simulink model "BPM_HA_Spin_sfun_xk"  (R2022b)
settings: configuration reference "ModelConfig_var" (kept outside this file)
InitFcn:
  | %% BUS initialization
  | Xabc.A = 0;
  | Xabc.B = 0;
  | Xabc.C = 0;
  | % -------------------------------------------------------------------------
  | Simulink.Bus.createObject(Xabc)
  | XabcBus = slBus1;
  | clear slBus1
  | 
  | %% Parameter Structure initialization
  | Motor_prm_init_bpm;
model workspace (MAT data in the model file):
  Mech_HAs_CF = 0
  Mech_HAs_J_drum = 0
  Mech_HAs_TR = 0
  Mech_HAs_damp = 0
  Mech_HAs_m_unb = 0
  Mech_HAs_r_unb = 0
  Mech_VAa_J_basket = 0
  Mech_VAa_J_impeller = 0
  Mech_VAa_basket_dens = 0
  Mech_VAa_basket_dia = 0
  Mech_VAa_belt_ratio = 0
  Mech_VAa_clothes_mass = 0
  Mech_VAa_gear_ratio = 0
  Mech_VAa_imp_dens = 0
  Mech_VAa_water_vol = 0
  Mech_VAs_D_r = 0
  Mech_VAs_I_zt = 0
  Mech_VAs_K = 2700
  Mech_VAs_T_f = 0
  Mech_VAs_belt_rat = 0
  Mech_VAs_d = 0
  Mech_VAs_e = 0
  Mech_VAs_m_b1 = 0
  Mech_VAs_m_b2 = 0
  Mech_VAs_m_d = 0
  Mech_VAs_m_t = 0
  Mech_VAs_m_u = 0
  Time_step = 0.0001
  Time_step_solver = 0
  bpm_B = 0
  bpm_Ipk = [0 1 2 3 4 5 6 7]
  bpm_Jrotor = 0
  bpm_Ld_0 = 0.02117
  bpm_Ld_a = [0.02117 0.02117 0.02117 0.02117 0.02117 0.02117 0.02117 0.02117]
  bpm_Loss_Power = [0 1 2 3 4 5 6 7]
  bpm_Loss_Speed = [0 1 2 3 4 5 6 7]
  bpm_Loss_flag = 1
  bpm_Loss_th = 10
  bpm_Lq_0 = 0.02117
  bpm_Lq_b = [0.02117 0.02117 0.02117 0.02117 0.02117 0.02117 0.02117 0.02117]
  bpm_Ls_sat_flag = 1
  bpm_NPP = 0
  bpm_PM_flux_h1_0 = 0
  bpm_PM_rotor_alpha = 0
  bpm_Rs_0 = 0
  bpm_Rs_stator_alpha = 0
  bpm_Rsa_aux = 0
  bpm_Rsb_aux = 0
  bpm_Rsc_aux = 0
  bpm_TR = 1
  bpm_Temp_rotor_0 = 0
  bpm_Temp_stator_0 = 0
libraries: bpm_dq_S_noH_D_RL_U_HA_Spin_xk x1
settings Model: ParameterArgumentNames=Mech_HAs_CF,Mech_HAs_J_drum,Mech_HAs_TR,Mech_HAs_damp,Mech_HAs_m_unb,Mech_HAs_r_unb,Mech_VAa_J_basket,Mech_VAa_J_impeller,Mech_VAa_basket_dens,Mech_VAa_basket_dia,Mech_VAa_belt_ratio,Mech_VAa_clothes_mass,Mech_VAa_gear_ratio,Mech_VAa_imp_dens,Mech_VAa_water_vol,Mech_VAs_D_r,Mech_VAs_I_zt,Mech_VAs_K,Mech_VAs_T_f,Mech_VAs_belt_rat,Mech_VAs_d,Mech_VAs_e,Mech_VAs_m_b1,Mech_VAs_m_b2,Mech_VAs_m_d,Mech_VAs_m_t,Mech_VAs_m_u,Time_step_solver,bpm_B,bpm_Ipk,bpm_Jrotor,bpm_Ld_0,bpm_Ld_a,bpm_Loss_Power,bpm_Loss_Speed,bpm_Loss_flag,bpm_Loss_th,bpm_Lq_0,bpm_Lq_b,bpm_Ls_sat_flag,bpm_NPP,bpm_PM_flux_h1_0,bpm_PM_rotor_alpha,bpm_Rs_0,bpm_Rs_stator_alpha,bpm_Rsa_aux,bpm_Rsb_aux,bpm_Rsc_aux,bpm_TR,bpm_Temp_rotor_0,bpm_Temp_stator_0  Creator=BEDNASA  LastModifiedBy=BEDNASA
settings ConfigSetRef: SourceName=ModelConfig_var  SourceLocation=Base Workspace

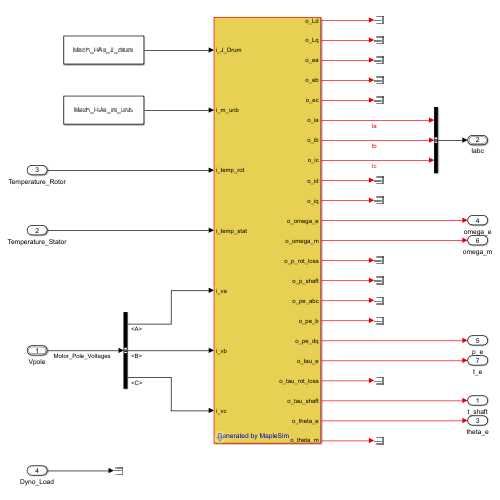
[thumbnail: Simulink's stored preview of the top-level diagram]
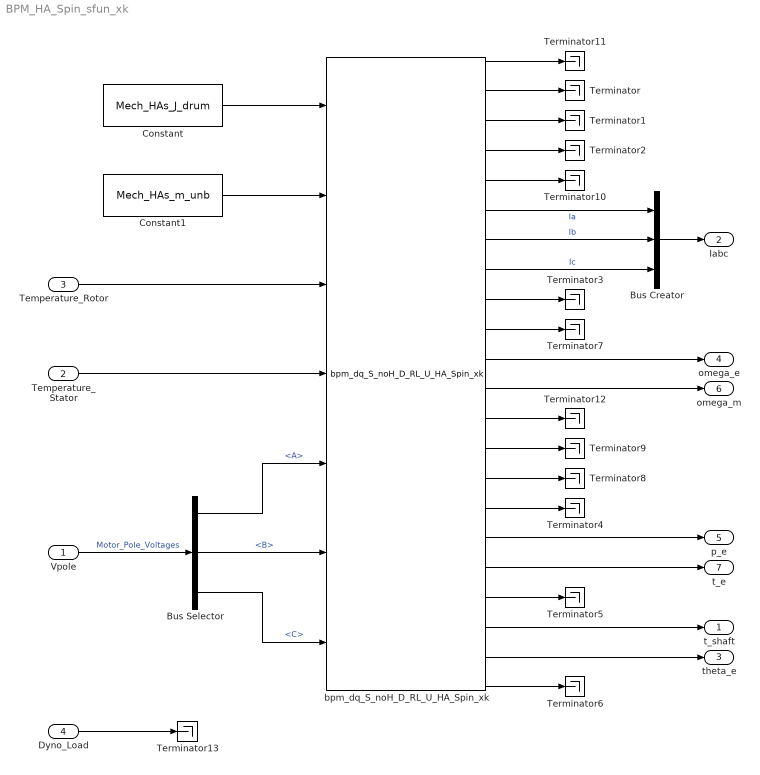
== system BPM_HA_Spin_sfun_xk ==
  Vpole : Inport  OutDataTypeStr=Bus: XabcBus
  Temperature_Stator : Inport  Port=2
  Temperature_Rotor : Inport  Port=3
  Dyno_Load : Inport  Port=4
  Bus Creator : BusCreator  Inputs=3
  Bus Selector : BusSelector  OutputSignals=A,B,C
  Constant : Constant  Value=Mech_HAs_J_drum
  Constant1 : Constant  Value=Mech_HAs_m_unb
  Terminator{,1..13} (14 alike) : Terminator
  bpm_dq_S_noH_D_RL_U_HA_Spin_xk : bpm_dq_S_noH_D_RL_U_HA_Spin_xk/bpm_dq_S_noH_D_RL_U_HA_Spin_xk  Description=Subsystem: bpm_dq_S_noH_D_RL_U_HA_Spin_xk  ic=[0., 0., 0., -0., 0.]  Par1=bpm_B  Par2=bpm_Ipk(1)  Par3=bpm_Ipk(2)  Par4=bpm_Ipk(3)  Par5=bpm_Ipk(4)  Par6=bpm_Ipk(5)  Par7=bpm_Ipk(6)  Par8=bpm_Ipk(7)  Par9=bpm_Ipk(8)  Par10=bpm_Jrotor  Par11=bpm_Ld_0  Par12=bpm_Ld_a(1)  Par13=bpm_Ld_a(2)  Par14=bpm_Ld_a(3)  Par15=bpm_Ld_a(4)  Par16=bpm_Ld_a(5)  Par17=bpm_Ld_a(6)  Par18=bpm_Ld_a(7)  Par19=bpm_Ld_a(8)  Par20=bpm_Lq_0  Par21=bpm_Lq_b(1)  Par22=bpm_Lq_b(2)  Par23=bpm_Lq_b(3)  Par24=bpm_Lq_b(4)  Par25=bpm_Lq_b(5)  Par26=bpm_Lq_b(6)  Par27=bpm_Lq_b(7)  Par28=bpm_Lq_b(8)  Par29=bpm_Ls_sat_flag  Par30=bpm_NPP  Par31=bpm_Loss_Power(1)  Par32=bpm_Loss_Power(2)  Par33=bpm_Loss_Power(3)  Par34=bpm_Loss_Power(4)  Par35=bpm_Loss_Power(5)  Par36=bpm_Loss_Power(6)  Par37=bpm_Loss_Power(7)  Par38=bpm_Loss_Power(8)  Par39=bpm_Loss_Speed(1)  Par40=bpm_Loss_Speed(2)  Par41=bpm_Loss_Speed(3)  Par42=bpm_Loss_Speed(4)  Par43=bpm_Loss_Speed(5)  Par44=bpm_Loss_Speed(6)  Par45=bpm_Loss_Speed(7)  Par46=bpm_Loss_Speed(8)  Par47=bpm_Loss_flag  Par48=bpm_Loss_th  Par49=bpm_Rs_0  Par50=bpm_Rsa_aux  Par51=bpm_Rsb_aux  Par52=bpm_Rsc_aux  Par53=bpm_Temp_rotor_0  Par54=bpm_Temp_stator_0  Par55=Time_step_solver  Par56=bpm_Rs_stator_alpha  Par57=bpm_PM_rotor_alpha  Par58=bpm_PM_flux_h1_0  Par59=Mech_HAs_CF  Par60=Mech_HAs_TR  Par61=Mech_HAs_damp  Par62=0.  Par63=0.  Par64=0.  Par65=-9.8  Par66=-1.  Par67=1.  MinStep=1/40  TimeStep_Solver=TimeSteps.ModelStep
  t_shaft : Outport  VectorParamsAs1DForOutWhenUnconnected=off
  Iabc : Outport  Port=2  OutDataTypeStr=Bus: XabcBus  VectorParamsAs1DForOutWhenUnconnected=off
  theta_e : Outport  Port=3  VectorParamsAs1DForOutWhenUnconnected=off
  omega_e : Outport  Port=4  VectorParamsAs1DForOutWhenUnconnected=off
  p_e : Outport  Port=5  VectorParamsAs1DForOutWhenUnconnected=off
  omega_m : Outport  Port=6  VectorParamsAs1DForOutWhenUnconnected=off
  t_e : Outport  Port=7  VectorParamsAs1DForOutWhenUnconnected=off
  wires:
  bpm_dq_S_noH_D_RL_U_HA_Spin_xk/2 -> Terminator/1
  bpm_dq_S_noH_D_RL_U_HA_Spin_xk/3 -> Terminator1/1
  bpm_dq_S_noH_D_RL_U_HA_Spin_xk/4 -> Terminator2/1
  bpm_dq_S_noH_D_RL_U_HA_Spin_xk/9 -> Terminator3/1
  bpm_dq_S_noH_D_RL_U_HA_Spin_xk/16 -> Terminator4/1
  bpm_dq_S_noH_D_RL_U_HA_Spin_xk/12 -> omega_m/1
  bpm_dq_S_noH_D_RL_U_HA_Spin_xk/11 -> omega_e/1
  bpm_dq_S_noH_D_RL_U_HA_Spin_xk/21 -> theta_e/1
  bpm_dq_S_noH_D_RL_U_HA_Spin_xk/18 -> t_e/1
  bpm_dq_S_noH_D_RL_U_HA_Spin_xk/20 -> t_shaft/1
  bpm_dq_S_noH_D_RL_U_HA_Spin_xk/19 -> Terminator5/1
  bpm_dq_S_noH_D_RL_U_HA_Spin_xk/22 -> Terminator6/1
  bpm_dq_S_noH_D_RL_U_HA_Spin_xk/10 -> Terminator7/1
  bpm_dq_S_noH_D_RL_U_HA_Spin_xk/17 -> p_e/1
  bpm_dq_S_noH_D_RL_U_HA_Spin_xk/15 -> Terminator8/1
  bpm_dq_S_noH_D_RL_U_HA_Spin_xk/5 -> Terminator10/1
  bpm_dq_S_noH_D_RL_U_HA_Spin_xk/1 -> Terminator11/1
  Bus Selector/3 -> bpm_dq_S_noH_D_RL_U_HA_Spin_xk/7  "<C>"
  Bus Selector/2 -> bpm_dq_S_noH_D_RL_U_HA_Spin_xk/6  "<B>"
  Vpole/1 -> Bus Selector/1  "Motor_Pole_Voltages"
  bpm_dq_S_noH_D_RL_U_HA_Spin_xk/7 -> Bus Creator/2  "Ib"
  Bus Creator/1 -> Iabc/1
  bpm_dq_S_noH_D_RL_U_HA_Spin_xk/6 -> Bus Creator/1  "Ia"
  bpm_dq_S_noH_D_RL_U_HA_Spin_xk/8 -> Bus Creator/3  "Ic"
  Bus Selector/1 -> bpm_dq_S_noH_D_RL_U_HA_Spin_xk/5  "<A>"
  bpm_dq_S_noH_D_RL_U_HA_Spin_xk/13 -> Terminator12/1
  bpm_dq_S_noH_D_RL_U_HA_Spin_xk/14 -> Terminator9/1
  Temperature_Stator/1 -> bpm_dq_S_noH_D_RL_U_HA_Spin_xk/4
  Temperature_Rotor/1 -> bpm_dq_S_noH_D_RL_U_HA_Spin_xk/3
  Dyno_Load/1 -> Terminator13/1
  Constant/1 -> bpm_dq_S_noH_D_RL_U_HA_Spin_xk/1
  Constant1/1 -> bpm_dq_S_noH_D_RL_U_HA_Spin_xk/2
